simulink model "sistemviza2"  (R2016a)
settings: Solver=VariableStepAuto  StartTime=0.0  StopTime=500  RelTol=1e-3
values from neighbouring files (symbols this model uses):
  Ag = 0.8    [Valori.m]
  dem = [0.917 1 0]    [Valori.m]
  Dg = 0    [Valori.m]
  Dg1 = 40    [Valori.m]
  Dg2 = 60    [Valori.m]
  Dg3 = 80    [Valori.m]
  Gb = 80    [Valori.m]
  kr = 2    [Valori.m]
  n = 0.109    [Valori.m]
  num = [1001.98 63.54 1]    [Valori.m]
  p1 = 0.029    [Valori.m]
  p2 = 0.029    [Valori.m]
  p3 = 0.00000783    (= 7.83e-06)    [Valori.m]
  tgmax = 40    [Valori.m]
  V = 120    [Valori.m]
  Xb = 0.0054    [Valori.m]
settings Model: Creator=carme  LastModifiedBy=midas

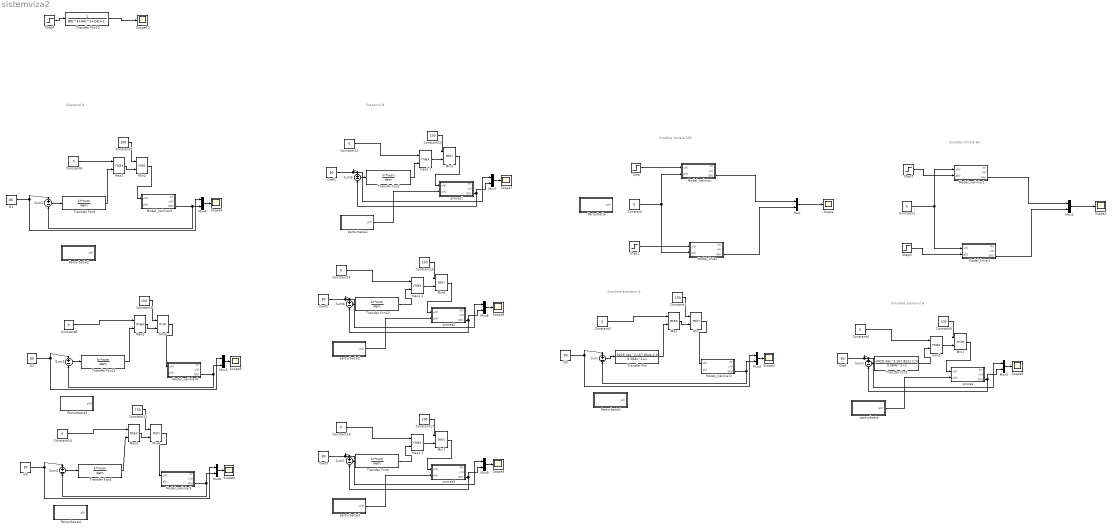
== system sistemviza2 ==
  note: Scenariul B
  note: Scenariul A
  note: Simulare scenariul B
  note: Simulare scenariul A
  note: Conditie initiala 80
  note: Conditie initiala 300
  Constant{,1..2,4,6,8,10,12,14,16} (10 alike) : Constant  Value=0
  Constant{3,5,7,9,11,13,15,17} (8 alike) : Constant  Value=100
  G{0..3} (4 alike) : Constant  Value=80
  Gref{,1..3} (4 alike) : Constant  Value=80
  Max{,1..3} (4 alike) : MinMax  Function=max  Inputs=2
  Min{,1..7} (8 alike) : MinMax  Inputs=2
  Model_liniar : Subsystem
  Model_liniar1 : Subsystem
  Model_neliniar : Subsystem
  Model_neliniar1 : Subsystem
  Model_neliniar2 : Subsystem
  Model_neliniar3 : Subsystem
  Model_neliniar4 : Subsystem
  Model_neliniar5 : Subsystem
  Mux{,1..9} (10 alike) : Mux  Inputs=2
  Perturbatie : Subsystem
  Perturbatie1 : Subsystem
  Perturbatie2 : Subsystem
  Perturbatie3 : Subsystem
  Perturbatie4 : Subsystem
  Scope{,1..10} (11 alike) : Scope
  Step{,1..4} (5 alike) : Step  SampleTime=0
  Sum{,1..7} (8 alike) : Sum  Inputs=+-
  Transfer Fcn : TransferFcn  Numerator=[-3029.34 -167.852 -2.32]  Denominator=[0.564 1 0]
  Transfer Fcn1 : TransferFcn  Numerator=[-3029.34 -167.852 -2.32]  Denominator=[0.564 1 0]
  Transfer Fcn10 : TransferFcn  Denominator=[80 84 24 1]
  Transfer Fcn{2,4,6,8,11..12} (6 alike) : TransferFcn  Numerator=kr*num  Denominator=dem
  max1 {,1..3} (4 alike) : MinMax  Function=max  Inputs=2
  perturbatie : Subsystem
  perturbatie1 : Subsystem
  perturbatie2 : Subsystem
  perturbatie3 : Subsystem
  proces : Subsystem
  proces1 : Subsystem
  proces2 : Subsystem
  proces3 : Subsystem
  wires:
  Mux/1 -> Scope/1
  Step/1 -> Model_neliniar/1(u(t))
  Constant/1 -> Model_neliniar/2(p(t)), Model_liniar/2(p(t))
  Step1/1 -> Model_liniar/1(u(t))
  Model_liniar/3(G(t)) -> Mux/2
  Model_neliniar/3(G(t)) -> Mux/1
  Mux1/1 -> Scope1/1
  Model_liniar1/3(G(t)) -> Mux1/2
  Model_neliniar1/3(G(t)) -> Mux1/1
  Constant1/1 -> Model_neliniar1/1(u(t)), Model_liniar1/1(u(t))
  Step3/1 -> Model_liniar1/2(p(t))
  Step2/1 -> Model_neliniar1/2(p(t))
  Mux2/1 -> Scope2/1
  Model_neliniar2/3(G(t)) -> Mux2/2, Sum/2
  G0/1 -> Mux2/1, Sum/1
  Constant2/1 -> Max/1
  Constant3/1 -> Min/1
  Max/1 -> Min/2
  Min/1 -> Model_neliniar2/1(u(t))
  Mux3/1 -> Scope3/1
  proces/3(G(t)) -> Mux3/2, Sum1/2
  Gref/1 -> Mux3/1, Sum1/1
  Constant4/1 -> "max1 "/1
  Constant5/1 -> Min1/1
  "max1 "/1 -> Min1/2
  Min1/1 -> proces/1(u(t))
  perturbatie/1(p(t)) -> proces/2(p(t))
  Transfer Fcn/1 -> Max/2
  Sum/1 -> Transfer Fcn/1
  Sum1/1 -> Transfer Fcn1/1
  Transfer Fcn1/1 -> "max1 "/2
  Mux5/1 -> Scope5/1
  Model_neliniar4/3(G(t)) -> Mux5/2, Sum3/2
  G2/1 -> Mux5/1, Sum3/1
  Constant8/1 -> Max2/1
  Constant9/1 -> Min3/1
  Max2/1 -> Min3/2
  Min3/1 -> Model_neliniar4/1(u(t))
  Mux6/1 -> Scope6/1
  Model_neliniar5/3(G(t)) -> Mux6/2, Sum4/2
  G3/1 -> Mux6/1, Sum4/1
  Constant10/1 -> Max3/1
  Constant11/1 -> Min4/1
  Max3/1 -> Min4/2
  Min4/1 -> Model_neliniar5/1(u(t))
  Transfer Fcn4/1 -> Max3/2
  Sum4/1 -> Transfer Fcn4/1
  Mux7/1 -> Scope7/1
  proces1/3(G(t)) -> Mux7/2, Sum5/2
  Gref1/1 -> Mux7/1, Sum5/1
  Constant12/1 -> max1 1/1
  Constant13/1 -> Min5/1
  max1 1/1 -> Min5/2
  Min5/1 -> proces1/1(u(t))
  perturbatie1/1(p(t)) -> proces1/2(p(t))
  Sum5/1 -> Transfer Fcn2/1
  Mux8/1 -> Scope8/1
  proces2/3(G(t)) -> Mux8/2, Sum6/2
  Gref2/1 -> Mux8/1, Sum6/1
  Constant14/1 -> max1 2/1
  Constant15/1 -> Min6/1
  max1 2/1 -> Min6/2
  Min6/1 -> proces2/1(u(t))
  perturbatie2/1(p(t)) -> proces2/2(p(t))
  Sum6/1 -> Transfer Fcn12/1
  Transfer Fcn12/1 -> max1 2/2
  Mux9/1 -> Scope9/1
  proces3/3(G(t)) -> Mux9/2, Sum7/2
  Gref3/1 -> Mux9/1, Sum7/1
  Constant16/1 -> max1 3/1
  Constant17/1 -> Min7/1
  max1 3/1 -> Min7/2
  Min7/1 -> proces3/1(u(t))
  perturbatie3/1(p(t)) -> proces3/2(p(t))
  Sum7/1 -> Transfer Fcn6/1
  Transfer Fcn6/1 -> max1 3/2
  Mux4/1 -> Scope4/1
  Model_neliniar3/3(G(t)) -> Sum2/2, Mux4/2
  G1/1 -> Mux4/1, Sum2/1
  Constant6/1 -> Max1/1
  Constant7/1 -> Min2/1
  Max1/1 -> Min2/2
  Min2/1 -> Model_neliniar3/1(u(t))
  Sum2/1 -> Transfer Fcn8/1
  Transfer Fcn8/1 -> Max1/2
  Transfer Fcn2/1 -> max1 1/2
  Transfer Fcn10/1 -> Scope10/1
  Step4/1 -> Transfer Fcn10/1
  Sum3/1 -> Transfer Fcn11/1
  Transfer Fcn11/1 -> Max2/2

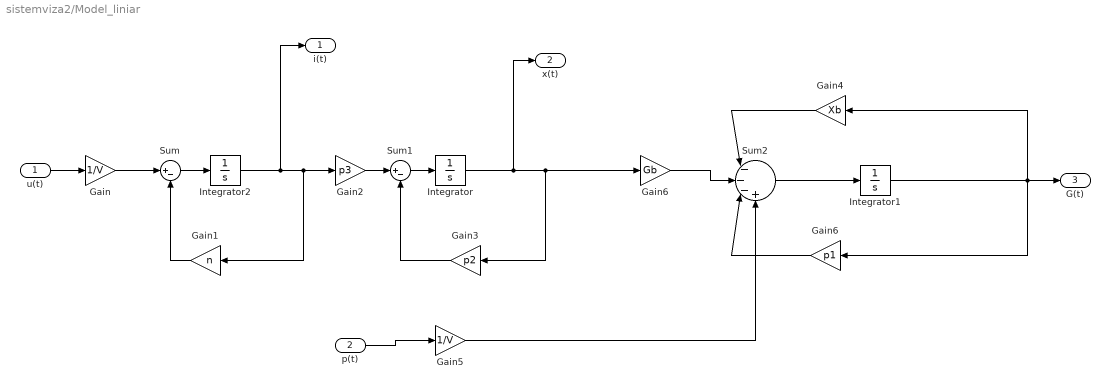
== system sistemviza2/Model_liniar ==
  u(t) : Inport
  p(t) : Inport  Port=2
  Gain : Gain  Gain=1/V
  Gain1 : Gain  Gain=n
  Gain2 : Gain  Gain=p3
  Gain3 : Gain  Gain=p2
  Gain4 : Gain  Gain=Xb
  Gain5 : Gain  Gain=1/V
  Gain6 : Gain  Gain=p1
  "Gain6 " : Gain  Gain=Gb
  Integrator : Integrator
  Integrator1 : Integrator  InitialCondition=300
  Integrator2 : Integrator
  Sum : Sum  Inputs=|+-
  Sum1 : Sum  Inputs=|+-
  Sum2 : Sum  Inputs=|---+
  i(t) : Outport
  x(t) : Outport  Port=2
  G(t) : Outport  Port=3
  wires:
  u(t)/1 -> Gain/1
  Gain/1 -> Sum/1
  Sum/1 -> Integrator2/1
  Integrator2/1 -> i(t)/1, Gain1/1, Gain2/1
  Gain2/1 -> Sum1/1
  Sum1/1 -> Integrator/1
  Gain1/1 -> Sum/2
  Gain3/1 -> Sum1/2
  Integrator/1 -> x(t)/1, Gain3/1, "Gain6 "/1
  p(t)/1 -> Gain5/1
  Gain5/1 -> Sum2/4
  "Gain6 "/1 -> Sum2/2
  Sum2/1 -> Integrator1/1
  Integrator1/1 -> Gain4/1, Gain6/1, G(t)/1
  Gain4/1 -> Sum2/1
  Gain6/1 -> Sum2/3

== system sistemviza2/Model_liniar1 ==
  u(t) : Inport
  p(t) : Inport  Port=2
  Gain : Gain  Gain=1/V
  Gain1 : Gain  Gain=n
  Gain2 : Gain  Gain=p3
  Gain3 : Gain  Gain=p2
  Gain4 : Gain  Gain=Xb
  Gain5 : Gain  Gain=1/V
  Gain6 : Gain  Gain=p1
  "Gain6 " : Gain  Gain=Gb
  Integrator : Integrator
  Integrator1 : Integrator  InitialCondition=80
  Integrator2 : Integrator
  Sum : Sum  Inputs=|+-
  Sum1 : Sum  Inputs=|+-
  Sum2 : Sum  Inputs=|---+
  i(t) : Outport
  x(t) : Outport  Port=2
  G(t) : Outport  Port=3
  wires:
  u(t)/1 -> Gain/1
  Gain/1 -> Sum/1
  Sum/1 -> Integrator2/1
  Integrator2/1 -> i(t)/1, Gain1/1, Gain2/1
  Gain2/1 -> Sum1/1
  Sum1/1 -> Integrator/1
  Gain1/1 -> Sum/2
  Gain3/1 -> Sum1/2
  Integrator/1 -> x(t)/1, Gain3/1, "Gain6 "/1
  p(t)/1 -> Gain5/1
  Gain5/1 -> Sum2/4
  "Gain6 "/1 -> Sum2/2
  Sum2/1 -> Integrator1/1
  Integrator1/1 -> Gain4/1, Gain6/1, G(t)/1
  Gain4/1 -> Sum2/1
  Gain6/1 -> Sum2/3

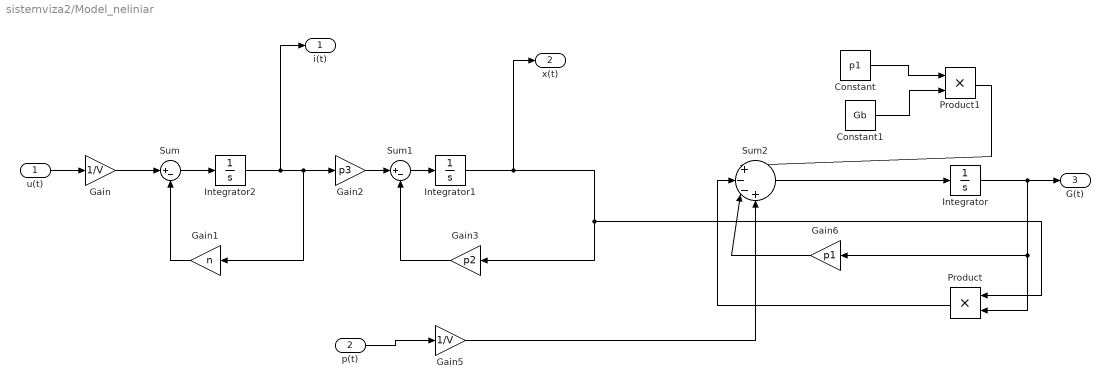
== system sistemviza2/Model_neliniar ==
  u(t) : Inport
  p(t) : Inport  Port=2
  Constant : Constant  Value=p1
  Constant1 : Constant  Value=Gb
  Gain : Gain  Gain=1/V
  Gain1 : Gain  Gain=n
  Gain2 : Gain  Gain=p3
  Gain3 : Gain  Gain=p2
  Gain5 : Gain  Gain=1/V
  Gain6 : Gain  Gain=p1
  Integrator : Integrator  InitialCondition=300
  Integrator1 : Integrator
  Integrator2 : Integrator
  Product : Product
  Product1 : Product
  Sum : Sum  Inputs=|+-
  Sum1 : Sum  Inputs=|+-
  Sum2 : Sum  Inputs=|+--+
  i(t) : Outport
  x(t) : Outport  Port=2
  G(t) : Outport  Port=3
  wires:
  u(t)/1 -> Gain/1
  Gain/1 -> Sum/1
  Sum/1 -> Integrator2/1
  Integrator2/1 -> i(t)/1, Gain1/1, Gain2/1
  Gain2/1 -> Sum1/1
  Sum1/1 -> Integrator1/1
  Gain1/1 -> Sum/2
  Gain3/1 -> Sum1/2
  Integrator1/1 -> x(t)/1, Product/1, Gain3/1
  p(t)/1 -> Gain5/1
  Gain5/1 -> Sum2/4
  Integrator/1 -> Product/2, Gain6/1, G(t)/1
  Gain6/1 -> Sum2/3
  Constant/1 -> Product1/1
  Constant1/1 -> Product1/2
  Product1/1 -> Sum2/1
  Product/1 -> Sum2/2
  Sum2/1 -> Integrator/1

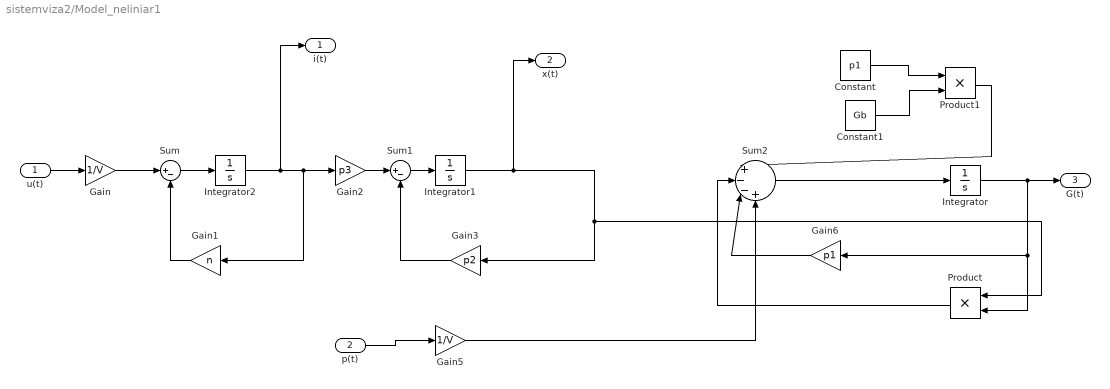
== system sistemviza2/Model_neliniar1 ==
  u(t) : Inport
  p(t) : Inport  Port=2
  Constant : Constant  Value=p1
  Constant1 : Constant  Value=Gb
  Gain : Gain  Gain=1/V
  Gain1 : Gain  Gain=n
  Gain2 : Gain  Gain=p3
  Gain3 : Gain  Gain=p2
  Gain5 : Gain  Gain=1/V
  Gain6 : Gain  Gain=p1
  Integrator : Integrator  InitialCondition=80
  Integrator1 : Integrator
  Integrator2 : Integrator
  Product : Product
  Product1 : Product
  Sum : Sum  Inputs=|+-
  Sum1 : Sum  Inputs=|+-
  Sum2 : Sum  Inputs=|+--+
  i(t) : Outport
  x(t) : Outport  Port=2
  G(t) : Outport  Port=3
  wires:
  u(t)/1 -> Gain/1
  Gain/1 -> Sum/1
  Sum/1 -> Integrator2/1
  Integrator2/1 -> i(t)/1, Gain1/1, Gain2/1
  Gain2/1 -> Sum1/1
  Sum1/1 -> Integrator1/1
  Gain1/1 -> Sum/2
  Gain3/1 -> Sum1/2
  Integrator1/1 -> x(t)/1, Product/1, Gain3/1
  p(t)/1 -> Gain5/1
  Gain5/1 -> Sum2/4
  Integrator/1 -> Product/2, Gain6/1, G(t)/1
  Gain6/1 -> Sum2/3
  Constant/1 -> Product1/1
  Constant1/1 -> Product1/2
  Product1/1 -> Sum2/1
  Product/1 -> Sum2/2
  Sum2/1 -> Integrator/1

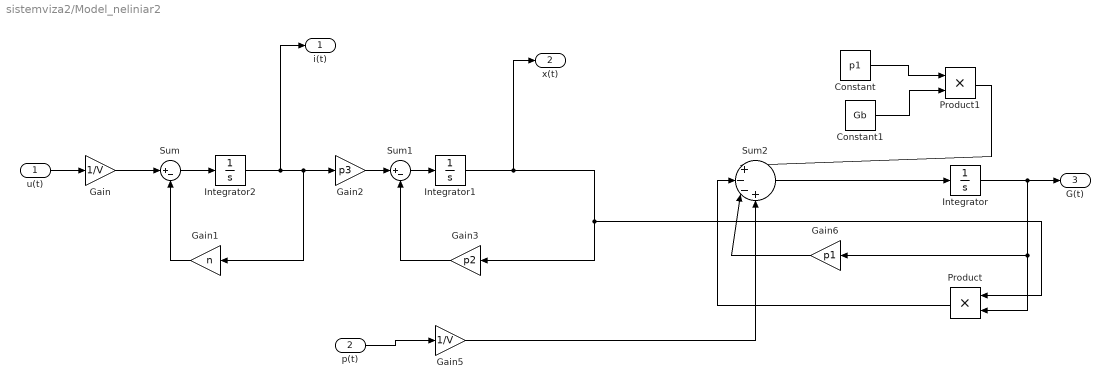
== system sistemviza2/Model_neliniar2 ==
  u(t) : Inport
  p(t) : Inport  Port=2
  Constant : Constant  Value=p1
  Constant1 : Constant  Value=Gb
  Gain : Gain  Gain=1/V
  Gain1 : Gain  Gain=n
  Gain2 : Gain  Gain=p3
  Gain3 : Gain  Gain=p2
  Gain5 : Gain  Gain=1/V
  Gain6 : Gain  Gain=p1
  Integrator : Integrator  InitialCondition=300
  Integrator1 : Integrator
  Integrator2 : Integrator
  Product : Product
  Product1 : Product
  Sum : Sum  Inputs=|+-
  Sum1 : Sum  Inputs=|+-
  Sum2 : Sum  Inputs=|+--+
  i(t) : Outport
  x(t) : Outport  Port=2
  G(t) : Outport  Port=3
  wires:
  u(t)/1 -> Gain/1
  Gain/1 -> Sum/1
  Sum/1 -> Integrator2/1
  Integrator2/1 -> i(t)/1, Gain1/1, Gain2/1
  Gain2/1 -> Sum1/1
  Sum1/1 -> Integrator1/1
  Gain1/1 -> Sum/2
  Gain3/1 -> Sum1/2
  Integrator1/1 -> x(t)/1, Product/1, Gain3/1
  p(t)/1 -> Gain5/1
  Gain5/1 -> Sum2/4
  Integrator/1 -> Product/2, Gain6/1, G(t)/1
  Gain6/1 -> Sum2/3
  Constant/1 -> Product1/1
  Constant1/1 -> Product1/2
  Product1/1 -> Sum2/1
  Product/1 -> Sum2/2
  Sum2/1 -> Integrator/1

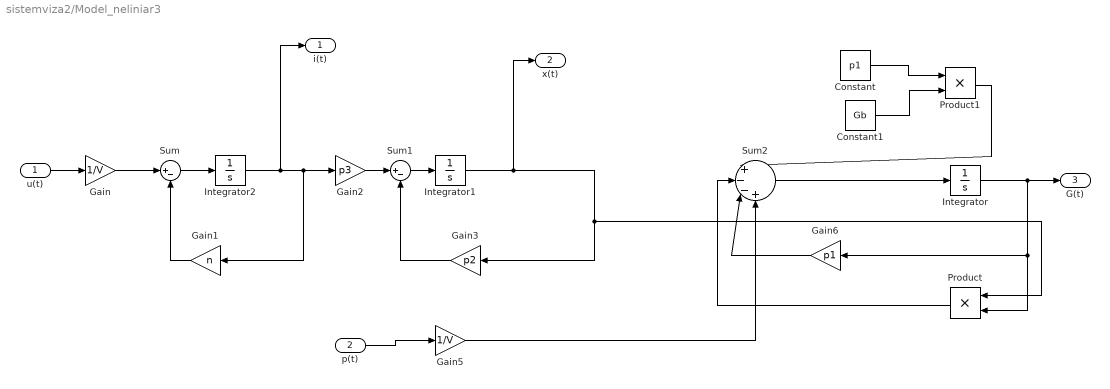
== system sistemviza2/Model_neliniar3 ==
  u(t) : Inport
  p(t) : Inport  Port=2
  Constant : Constant  Value=p1
  Constant1 : Constant  Value=Gb
  Gain : Gain  Gain=1/V
  Gain1 : Gain  Gain=n
  Gain2 : Gain  Gain=p3
  Gain3 : Gain  Gain=p2
  Gain5 : Gain  Gain=1/V
  Gain6 : Gain  Gain=p1
  Integrator : Integrator  InitialCondition=120
  Integrator1 : Integrator
  Integrator2 : Integrator
  Product : Product
  Product1 : Product
  Sum : Sum  Inputs=|+-
  Sum1 : Sum  Inputs=|+-
  Sum2 : Sum  Inputs=|+--+
  i(t) : Outport
  x(t) : Outport  Port=2
  G(t) : Outport  Port=3
  wires:
  u(t)/1 -> Gain/1
  Gain/1 -> Sum/1
  Sum/1 -> Integrator2/1
  Integrator2/1 -> i(t)/1, Gain1/1, Gain2/1
  Gain2/1 -> Sum1/1
  Sum1/1 -> Integrator1/1
  Gain1/1 -> Sum/2
  Gain3/1 -> Sum1/2
  Integrator1/1 -> x(t)/1, Product/1, Gain3/1
  p(t)/1 -> Gain5/1
  Gain5/1 -> Sum2/4
  Integrator/1 -> Product/2, Gain6/1, G(t)/1
  Gain6/1 -> Sum2/3
  Constant/1 -> Product1/1
  Constant1/1 -> Product1/2
  Product1/1 -> Sum2/1
  Product/1 -> Sum2/2
  Sum2/1 -> Integrator/1

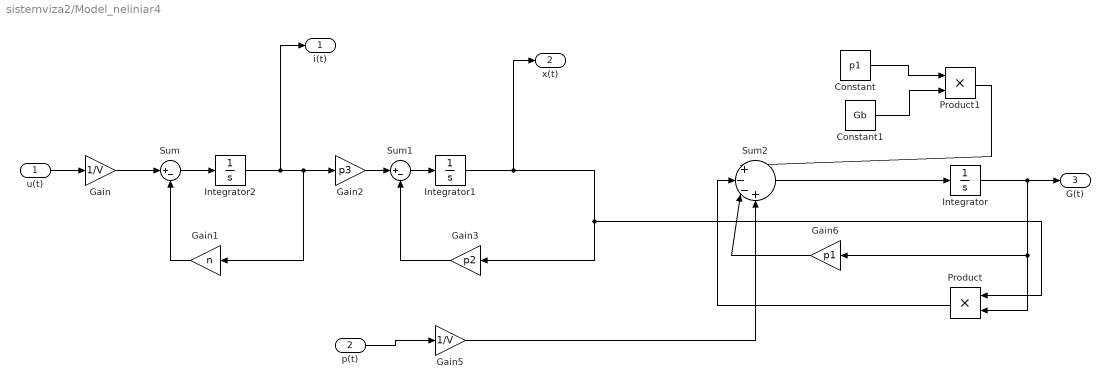
== system sistemviza2/Model_neliniar4 ==
  u(t) : Inport
  p(t) : Inport  Port=2
  Constant : Constant  Value=p1
  Constant1 : Constant  Value=Gb
  Gain : Gain  Gain=1/V
  Gain1 : Gain  Gain=n
  Gain2 : Gain  Gain=p3
  Gain3 : Gain  Gain=p2
  Gain5 : Gain  Gain=1/V
  Gain6 : Gain  Gain=p1
  Integrator : Integrator  InitialCondition=200
  Integrator1 : Integrator
  Integrator2 : Integrator
  Product : Product
  Product1 : Product
  Sum : Sum  Inputs=|+-
  Sum1 : Sum  Inputs=|+-
  Sum2 : Sum  Inputs=|+--+
  i(t) : Outport
  x(t) : Outport  Port=2
  G(t) : Outport  Port=3
  wires:
  u(t)/1 -> Gain/1
  Gain/1 -> Sum/1
  Sum/1 -> Integrator2/1
  Integrator2/1 -> i(t)/1, Gain1/1, Gain2/1
  Gain2/1 -> Sum1/1
  Sum1/1 -> Integrator1/1
  Gain1/1 -> Sum/2
  Gain3/1 -> Sum1/2
  Integrator1/1 -> x(t)/1, Product/1, Gain3/1
  p(t)/1 -> Gain5/1
  Gain5/1 -> Sum2/4
  Integrator/1 -> Product/2, Gain6/1, G(t)/1
  Gain6/1 -> Sum2/3
  Constant/1 -> Product1/1
  Constant1/1 -> Product1/2
  Product1/1 -> Sum2/1
  Product/1 -> Sum2/2
  Sum2/1 -> Integrator/1

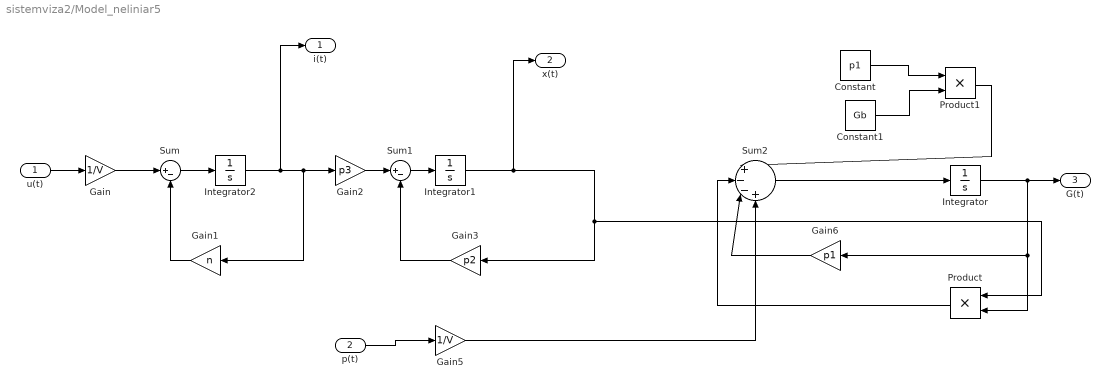
== system sistemviza2/Model_neliniar5 ==
  u(t) : Inport
  p(t) : Inport  Port=2
  Constant : Constant  Value=p1
  Constant1 : Constant  Value=Gb
  Gain : Gain  Gain=1/V
  Gain1 : Gain  Gain=n
  Gain2 : Gain  Gain=p3
  Gain3 : Gain  Gain=p2
  Gain5 : Gain  Gain=1/V
  Gain6 : Gain  Gain=p1
  Integrator : Integrator  InitialCondition=300
  Integrator1 : Integrator
  Integrator2 : Integrator
  Product : Product
  Product1 : Product
  Sum : Sum  Inputs=|+-
  Sum1 : Sum  Inputs=|+-
  Sum2 : Sum  Inputs=|+--+
  i(t) : Outport
  x(t) : Outport  Port=2
  G(t) : Outport  Port=3
  wires:
  u(t)/1 -> Gain/1
  Gain/1 -> Sum/1
  Sum/1 -> Integrator2/1
  Integrator2/1 -> i(t)/1, Gain1/1, Gain2/1
  Gain2/1 -> Sum1/1
  Sum1/1 -> Integrator1/1
  Gain1/1 -> Sum/2
  Gain3/1 -> Sum1/2
  Integrator1/1 -> x(t)/1, Product/1, Gain3/1
  p(t)/1 -> Gain5/1
  Gain5/1 -> Sum2/4
  Integrator/1 -> Product/2, Gain6/1, G(t)/1
  Gain6/1 -> Sum2/3
  Constant/1 -> Product1/1
  Constant1/1 -> Product1/2
  Product1/1 -> Sum2/1
  Product/1 -> Sum2/2
  Sum2/1 -> Integrator/1

== system sistemviza2/Perturbatie ==
  Ag : Constant  Value=Ag
  "Clock " : Clock
  Dg : Constant  Value=Dg
  Divide : Product  Inputs=*/
  Divide1 : Product  Inputs=*/
  Gain : Gain  Gain=-1
  Math Function : Math  SaturateOnIntegerOverflow=on
  Product : Product  Inputs=4
  Product1 : Product
  tg,max : Constant  Value=tgmax
  p(t) : Outport
  wires:
  Dg/1 -> Product/1
  Ag/1 -> Product/2
  Math Function/1 -> Product/3
  "Clock "/1 -> Product/4, Gain/1
  tg,max/1 -> Divide/2, Product1/2, Product1/1
  Divide/1 -> Math Function/1
  Gain/1 -> Divide/1
  Product1/1 -> Divide1/2
  Divide1/1 -> p(t)/1
  Product/1 -> Divide1/1

== system sistemviza2/Perturbatie1 ==
  Ag : Constant  Value=Ag
  "Clock " : Clock
  Dg : Constant  Value=Dg
  Divide : Product  Inputs=*/
  Divide1 : Product  Inputs=*/
  Gain : Gain  Gain=-1
  Math Function : Math  SaturateOnIntegerOverflow=on
  Product : Product  Inputs=4
  Product1 : Product
  tg,max : Constant  Value=tgmax
  p(t) : Outport
  wires:
  Dg/1 -> Product/1
  Ag/1 -> Product/2
  Math Function/1 -> Product/3
  "Clock "/1 -> Product/4, Gain/1
  tg,max/1 -> Divide/2, Product1/2, Product1/1
  Divide/1 -> Math Function/1
  Gain/1 -> Divide/1
  Product1/1 -> Divide1/2
  Divide1/1 -> p(t)/1
  Product/1 -> Divide1/1

== system sistemviza2/Perturbatie2 ==
  Ag : Constant  Value=Ag
  "Clock " : Clock
  Dg : Constant  Value=Dg
  Divide : Product  Inputs=*/
  Divide1 : Product  Inputs=*/
  Gain : Gain  Gain=-1
  Math Function : Math  SaturateOnIntegerOverflow=on
  Product : Product  Inputs=4
  Product1 : Product
  tg,max : Constant  Value=tgmax
  p(t) : Outport
  wires:
  Dg/1 -> Product/1
  Ag/1 -> Product/2
  Math Function/1 -> Product/3
  "Clock "/1 -> Product/4, Gain/1
  tg,max/1 -> Divide/2, Product1/2, Product1/1
  Divide/1 -> Math Function/1
  Gain/1 -> Divide/1
  Product1/1 -> Divide1/2
  Divide1/1 -> p(t)/1
  Product/1 -> Divide1/1

== system sistemviza2/Perturbatie3 ==
  Ag : Constant  Value=Ag
  "Clock " : Clock
  Dg : Constant  Value=Dg
  Divide : Product  Inputs=*/
  Divide1 : Product  Inputs=*/
  Gain : Gain  Gain=-1
  Math Function : Math  SaturateOnIntegerOverflow=on
  Product : Product  Inputs=4
  Product1 : Product
  tg,max : Constant  Value=tgmax
  p(t) : Outport
  wires:
  Dg/1 -> Product/1
  Ag/1 -> Product/2
  Math Function/1 -> Product/3
  "Clock "/1 -> Product/4, Gain/1
  tg,max/1 -> Divide/2, Product1/2, Product1/1
  Divide/1 -> Math Function/1
  Gain/1 -> Divide/1
  Product1/1 -> Divide1/2
  Divide1/1 -> p(t)/1
  Product/1 -> Divide1/1

== system sistemviza2/Perturbatie4 ==
  Ag : Constant  Value=Ag
  "Clock " : Clock
  Dg : Constant  Value=Dg
  Divide : Product  Inputs=*/
  Divide1 : Product  Inputs=*/
  Gain : Gain  Gain=-1
  Math Function : Math  SaturateOnIntegerOverflow=on
  Product : Product  Inputs=4
  Product1 : Product
  tg,max : Constant  Value=tgmax
  p(t) : Outport
  wires:
  Dg/1 -> Product/1
  Ag/1 -> Product/2
  Math Function/1 -> Product/3
  "Clock "/1 -> Product/4, Gain/1
  tg,max/1 -> Divide/2, Product1/2, Product1/1
  Divide/1 -> Math Function/1
  Gain/1 -> Divide/1
  Product1/1 -> Divide1/2
  Divide1/1 -> p(t)/1
  Product/1 -> Divide1/1

== system sistemviza2/perturbatie ==
  Ag : Constant  Value=Ag
  "Clock " : Clock
  Dg : Constant  Value=Dg
  Divide : Product  Inputs=*/
  Divide1 : Product  Inputs=*/
  Gain : Gain  Gain=-1
  Math Function : Math  SaturateOnIntegerOverflow=on
  Product : Product  Inputs=4
  Product1 : Product
  tg,max : Constant  Value=tgmax
  p(t) : Outport
  wires:
  Dg/1 -> Product/1
  Ag/1 -> Product/2
  Math Function/1 -> Product/3
  "Clock "/1 -> Product/4, Gain/1
  tg,max/1 -> Divide/2, Product1/2, Product1/1
  Divide/1 -> Math Function/1
  Gain/1 -> Divide/1
  Product1/1 -> Divide1/2
  Divide1/1 -> p(t)/1
  Product/1 -> Divide1/1

== system sistemviza2/perturbatie1 ==
  Ag : Constant  Value=Ag
  "Clock " : Clock
  Dg : Constant  Value=Dg1
  Divide : Product  Inputs=*/
  Divide1 : Product  Inputs=*/
  Gain : Gain  Gain=-1
  Math Function : Math  SaturateOnIntegerOverflow=on
  Product : Product  Inputs=4
  Product1 : Product
  tg,max : Constant  Value=tgmax
  p(t) : Outport
  wires:
  Dg/1 -> Product/1
  Ag/1 -> Product/2
  Math Function/1 -> Product/3
  "Clock "/1 -> Product/4, Gain/1
  tg,max/1 -> Divide/2, Product1/2, Product1/1
  Divide/1 -> Math Function/1
  Gain/1 -> Divide/1
  Product1/1 -> Divide1/2
  Divide1/1 -> p(t)/1
  Product/1 -> Divide1/1

== system sistemviza2/perturbatie2 ==
  Ag : Constant  Value=Ag
  "Clock " : Clock
  Dg : Constant  Value=Dg2
  Divide : Product  Inputs=*/
  Divide1 : Product  Inputs=*/
  Gain : Gain  Gain=-1
  Math Function : Math  SaturateOnIntegerOverflow=on
  Product : Product  Inputs=4
  Product1 : Product
  tg,max : Constant  Value=tgmax
  p(t) : Outport
  wires:
  Dg/1 -> Product/1
  Ag/1 -> Product/2
  Math Function/1 -> Product/3
  "Clock "/1 -> Product/4, Gain/1
  tg,max/1 -> Divide/2, Product1/2, Product1/1
  Divide/1 -> Math Function/1
  Gain/1 -> Divide/1
  Product1/1 -> Divide1/2
  Divide1/1 -> p(t)/1
  Product/1 -> Divide1/1

== system sistemviza2/perturbatie3 ==
  Ag : Constant  Value=Ag
  "Clock " : Clock
  Dg : Constant  Value=Dg3
  Divide : Product  Inputs=*/
  Divide1 : Product  Inputs=*/
  Gain : Gain  Gain=-1
  Math Function : Math  SaturateOnIntegerOverflow=on
  Product : Product  Inputs=4
  Product1 : Product
  tg,max : Constant  Value=tgmax
  p(t) : Outport
  wires:
  Dg/1 -> Product/1
  Ag/1 -> Product/2
  Math Function/1 -> Product/3
  "Clock "/1 -> Product/4, Gain/1
  tg,max/1 -> Divide/2, Product1/2, Product1/1
  Divide/1 -> Math Function/1
  Gain/1 -> Divide/1
  Product1/1 -> Divide1/2
  Divide1/1 -> p(t)/1
  Product/1 -> Divide1/1

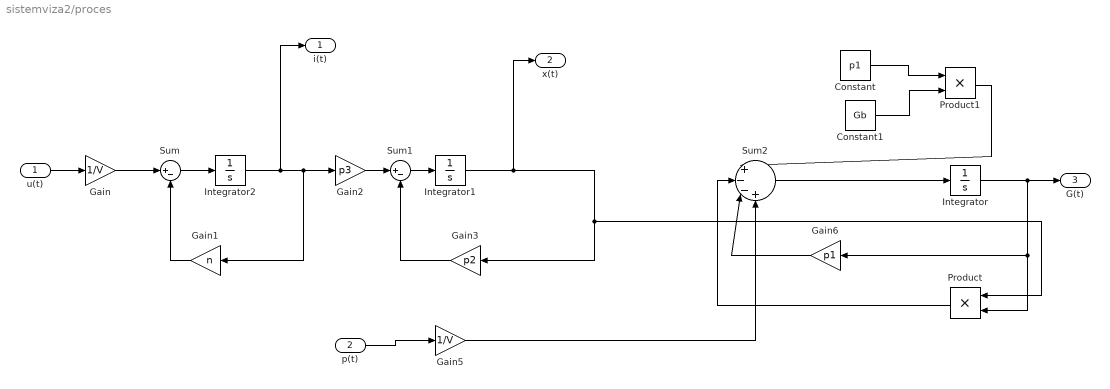
== system sistemviza2/proces ==
  u(t) : Inport
  p(t) : Inport  Port=2
  Constant : Constant  Value=p1
  Constant1 : Constant  Value=Gb
  Gain : Gain  Gain=1/V
  Gain1 : Gain  Gain=n
  Gain2 : Gain  Gain=p3
  Gain3 : Gain  Gain=p2
  Gain5 : Gain  Gain=1/V
  Gain6 : Gain  Gain=p1
  Integrator : Integrator  InitialCondition=80
  Integrator1 : Integrator
  Integrator2 : Integrator
  Product : Product
  Product1 : Product
  Sum : Sum  Inputs=|+-
  Sum1 : Sum  Inputs=|+-
  Sum2 : Sum  Inputs=|+--+
  i(t) : Outport
  x(t) : Outport  Port=2
  G(t) : Outport  Port=3
  wires:
  u(t)/1 -> Gain/1
  Gain/1 -> Sum/1
  Sum/1 -> Integrator2/1
  Integrator2/1 -> i(t)/1, Gain1/1, Gain2/1
  Gain2/1 -> Sum1/1
  Sum1/1 -> Integrator1/1
  Gain1/1 -> Sum/2
  Gain3/1 -> Sum1/2
  Integrator1/1 -> x(t)/1, Product/1, Gain3/1
  p(t)/1 -> Gain5/1
  Gain5/1 -> Sum2/4
  Integrator/1 -> Product/2, Gain6/1, G(t)/1
  Gain6/1 -> Sum2/3
  Constant/1 -> Product1/1
  Constant1/1 -> Product1/2
  Product1/1 -> Sum2/1
  Product/1 -> Sum2/2
  Sum2/1 -> Integrator/1

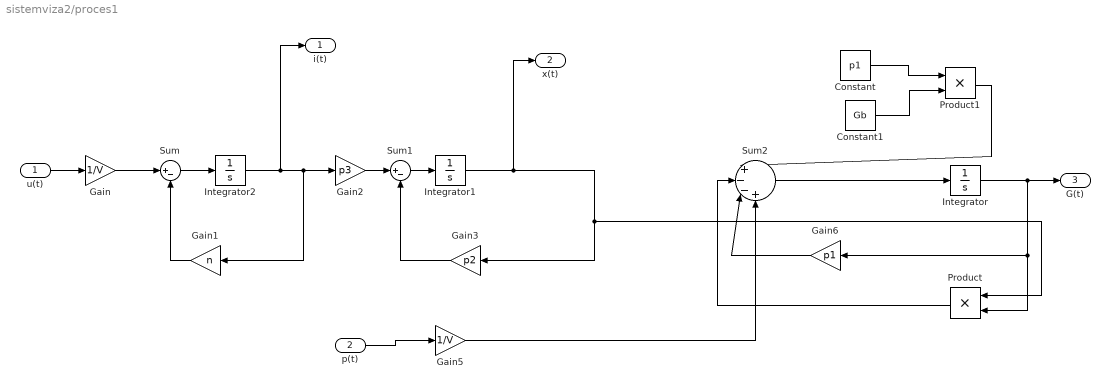
== system sistemviza2/proces1 ==
  u(t) : Inport
  p(t) : Inport  Port=2
  Constant : Constant  Value=p1
  Constant1 : Constant  Value=Gb
  Gain : Gain  Gain=1/V
  Gain1 : Gain  Gain=n
  Gain2 : Gain  Gain=p3
  Gain3 : Gain  Gain=p2
  Gain5 : Gain  Gain=1/V
  Gain6 : Gain  Gain=p1
  Integrator : Integrator  InitialCondition=80
  Integrator1 : Integrator
  Integrator2 : Integrator
  Product : Product
  Product1 : Product
  Sum : Sum  Inputs=|+-
  Sum1 : Sum  Inputs=|+-
  Sum2 : Sum  Inputs=|+--+
  i(t) : Outport
  x(t) : Outport  Port=2
  G(t) : Outport  Port=3
  wires:
  u(t)/1 -> Gain/1
  Gain/1 -> Sum/1
  Sum/1 -> Integrator2/1
  Integrator2/1 -> i(t)/1, Gain1/1, Gain2/1
  Gain2/1 -> Sum1/1
  Sum1/1 -> Integrator1/1
  Gain1/1 -> Sum/2
  Gain3/1 -> Sum1/2
  Integrator1/1 -> x(t)/1, Product/1, Gain3/1
  p(t)/1 -> Gain5/1
  Gain5/1 -> Sum2/4
  Integrator/1 -> Product/2, Gain6/1, G(t)/1
  Gain6/1 -> Sum2/3
  Constant/1 -> Product1/1
  Constant1/1 -> Product1/2
  Product1/1 -> Sum2/1
  Product/1 -> Sum2/2
  Sum2/1 -> Integrator/1

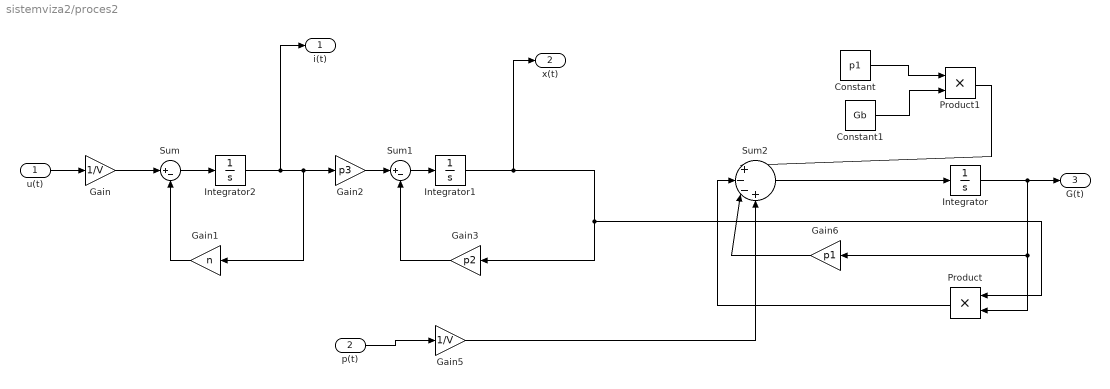
== system sistemviza2/proces2 ==
  u(t) : Inport
  p(t) : Inport  Port=2
  Constant : Constant  Value=p1
  Constant1 : Constant  Value=Gb
  Gain : Gain  Gain=1/V
  Gain1 : Gain  Gain=n
  Gain2 : Gain  Gain=p3
  Gain3 : Gain  Gain=p2
  Gain5 : Gain  Gain=1/V
  Gain6 : Gain  Gain=p1
  Integrator : Integrator  InitialCondition=80
  Integrator1 : Integrator
  Integrator2 : Integrator
  Product : Product
  Product1 : Product
  Sum : Sum  Inputs=|+-
  Sum1 : Sum  Inputs=|+-
  Sum2 : Sum  Inputs=|+--+
  i(t) : Outport
  x(t) : Outport  Port=2
  G(t) : Outport  Port=3
  wires:
  u(t)/1 -> Gain/1
  Gain/1 -> Sum/1
  Sum/1 -> Integrator2/1
  Integrator2/1 -> i(t)/1, Gain1/1, Gain2/1
  Gain2/1 -> Sum1/1
  Sum1/1 -> Integrator1/1
  Gain1/1 -> Sum/2
  Gain3/1 -> Sum1/2
  Integrator1/1 -> x(t)/1, Product/1, Gain3/1
  p(t)/1 -> Gain5/1
  Gain5/1 -> Sum2/4
  Integrator/1 -> Product/2, Gain6/1, G(t)/1
  Gain6/1 -> Sum2/3
  Constant/1 -> Product1/1
  Constant1/1 -> Product1/2
  Product1/1 -> Sum2/1
  Product/1 -> Sum2/2
  Sum2/1 -> Integrator/1

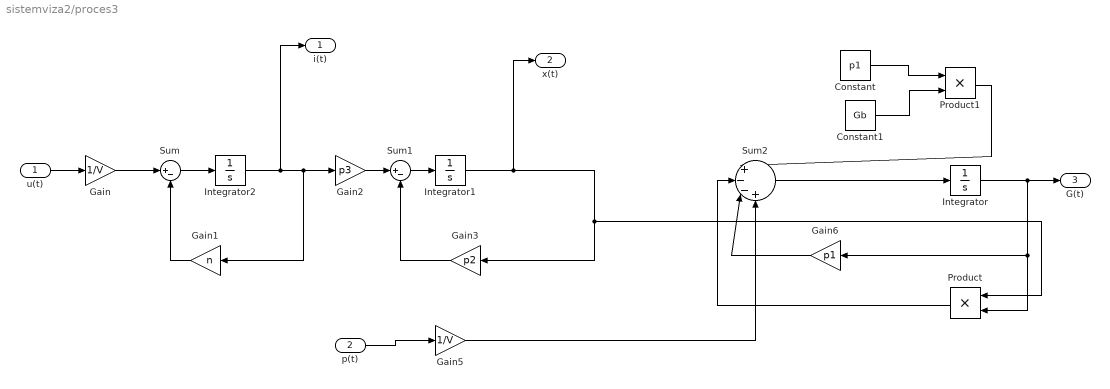
== system sistemviza2/proces3 ==
  u(t) : Inport
  p(t) : Inport  Port=2
  Constant : Constant  Value=p1
  Constant1 : Constant  Value=Gb
  Gain : Gain  Gain=1/V
  Gain1 : Gain  Gain=n
  Gain2 : Gain  Gain=p3
  Gain3 : Gain  Gain=p2
  Gain5 : Gain  Gain=1/V
  Gain6 : Gain  Gain=p1
  Integrator : Integrator  InitialCondition=80
  Integrator1 : Integrator
  Integrator2 : Integrator
  Product : Product
  Product1 : Product
  Sum : Sum  Inputs=|+-
  Sum1 : Sum  Inputs=|+-
  Sum2 : Sum  Inputs=|+--+
  i(t) : Outport
  x(t) : Outport  Port=2
  G(t) : Outport  Port=3
  wires:
  u(t)/1 -> Gain/1
  Gain/1 -> Sum/1
  Sum/1 -> Integrator2/1
  Integrator2/1 -> i(t)/1, Gain1/1, Gain2/1
  Gain2/1 -> Sum1/1
  Sum1/1 -> Integrator1/1
  Gain1/1 -> Sum/2
  Gain3/1 -> Sum1/2
  Integrator1/1 -> x(t)/1, Product/1, Gain3/1
  p(t)/1 -> Gain5/1
  Gain5/1 -> Sum2/4
  Integrator/1 -> Product/2, Gain6/1, G(t)/1
  Gain6/1 -> Sum2/3
  Constant/1 -> Product1/1
  Constant1/1 -> Product1/2
  Product1/1 -> Sum2/1
  Product/1 -> Sum2/2
  Sum2/1 -> Integrator/1
